simulink model "truxal_"  (R2020b)
settings: Solver=VariableStepAuto  StartTime=0.0  StopTime=5  RelTol=1e-3
values from neighbouring files (symbols this model uses):
  gc = tf([q21 q11 q01],[p21 p11 p01 0])    [ejemplo_6.m]    (also in truxal.m = N/(Gp*(D-N*H)))
settings Model: Creator=cmparedes  LastModifiedBy=Acer
settings SFSimCC: CustomCodeUndefinedFunction=UseInterfaceOnly

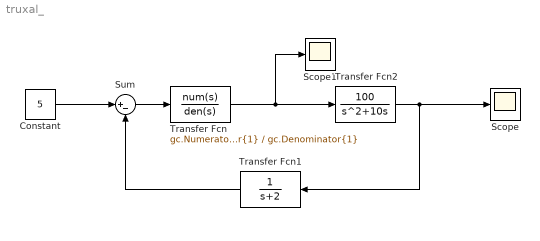
== system truxal_ ==
  Constant : Constant  Value=5
  Scope : Scope
  Scope1 : Scope
  Sum : Sum  Inputs=|+-
  Transfer Fcn : TransferFcn  Numerator=gc.Numerator{1}  Denominator=gc.Denominator{1}
  Transfer Fcn1 : TransferFcn  Denominator=[1 2]
  Transfer Fcn2 : TransferFcn  Numerator=[100]  Denominator=[1 10 0]
  wires:
  Sum/1 -> Transfer Fcn/1
  Transfer Fcn/1 -> Scope1/1, Transfer Fcn2/1
  Transfer Fcn2/1 -> Scope/1, Transfer Fcn1/1
  Transfer Fcn1/1 -> Sum/2
  Constant/1 -> Sum/1
